simulink model "Task3"  (R2021b)
settings: Solver=VariableStepAuto  StartTime=0.0  StopTime=10.0  RelTol=1e-3
settings Model: Creator=mluser  LastModifiedBy=mluser

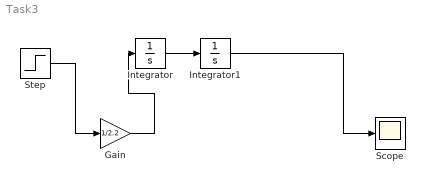
== system Task3 ==
  Gain : Gain  Gain=1/2.2
  Integrator : Integrator
  Integrator1 : Integrator
  Scope : Scope
  Step : Step  SampleTime=0
  wires:
  Integrator/1 -> Integrator1/1
  Integrator1/1 -> Scope/1
  Step/1 -> Gain/1
  Gain/1 -> Integrator/1
